simulink model "Telerobotic_System"  (R2020a)
settings: Solver=VariableStepAuto  StartTime=0.0  StopTime=10.0  RelTol=1e-3
values from neighbouring files (symbols this model uses):
  B = 1 / k_m    (= 0.0517063081696)    [Teleop_parameters.m]    (also in base.mat; base_no_attrito.mat = 0; ci_siamo.mat; force_control.mat)
  Be = 5    [Teleop_parameters.m]    (also in base.mat = 0.5; base_no_attrito.mat = 0.5; ci_siamo.mat; force_control.mat = 0.5)
  Bh = 0.02    [Teleop_parameters.m]    (also in base.mat; base_no_attrito.mat; ci_siamo.mat; force_control.mat)
  Fc_h = 5    [Teleop_parameters.m]    (also in base.mat; base_no_attrito.mat; ci_siamo.mat; force_control.mat)
  J = tau_m / k_m    (= 0.0629265770424)    [Teleop_parameters.m]    (also in base.mat; base_no_attrito.mat; ci_siamo.mat; force_control.mat)
  J_r = J + J * 0.5    (= 0.0943898655636)    [Teleop_parameters.m]    (also in base.mat; base_no_attrito.mat; ci_siamo.mat = 0.0629265770424; force_control.mat)
  Jh = 0.02    [Teleop_parameters.m]    (also in base.mat; base_no_attrito.mat; ci_siamo.mat; force_control.mat)
  k_m = 19.34    [Teleop_parameters.m]    (also in base.mat; base_no_attrito.mat; ci_siamo.mat; force_control.mat)
  k_s = 19.34    [Teleop_parameters.m]    (also in base.mat; base_no_attrito.mat; ci_siamo.mat; force_control.mat)
  Kc2v_m = 2    [Teleop_parameters.m]    (also in base.mat; base_no_attrito.mat; ci_siamo.mat; force_control.mat)
  Kc2v_s = 2    [Teleop_parameters.m]    (also in base.mat; base_no_attrito.mat; ci_siamo.mat; force_control.mat)
  Kd_h = 1    [Teleop_parameters.m]    (also in base.mat; base_no_attrito.mat; ci_siamo.mat = 10; force_control.mat)
  Kd_m = 1    [Teleop_parameters.m]    (also in base.mat; base_no_attrito.mat; ci_siamo.mat = 0.005; force_control.mat)
  Ke = 10    [Teleop_parameters.m]    (also in base.mat; base_no_attrito.mat; ci_siamo.mat; force_control.mat)
  Kp_h = 1.2    [Teleop_parameters.m]    (also in base.mat; base_no_attrito.mat; ci_siamo.mat = 10; force_control.mat)
  Kp_m = 1    [Teleop_parameters.m]    (also in base.mat; base_no_attrito.mat; ci_siamo.mat = 0.01; force_control.mat)
  Kt2c_m = 1.182    [Teleop_parameters.m]    (also in base.mat; base_no_attrito.mat; ci_siamo.mat; force_control.mat)
  Kt2c_s = 1.182    [Teleop_parameters.m]    (also in base.mat; base_no_attrito.mat; ci_siamo.mat; force_control.mat)
  Kv_fc = 30    [Teleop_parameters.m]    (also in base.mat = 0; base_no_attrito.mat = 0; ci_siamo.mat = 10; force_control.mat)
  lArm_m = 0.1    [Teleop_parameters.m]    (also in base.mat; base_no_attrito.mat; ci_siamo.mat; force_control.mat)
  lArm_s = 0.1    [Teleop_parameters.m]    (also in base.mat; base_no_attrito.mat; ci_siamo.mat; force_control.mat)
  maxCurrent_m = 4.5    [Teleop_parameters.m]    (also in base.mat; base_no_attrito.mat; ci_siamo.mat; force_control.mat)
  maxCurrent_s = 4.5    [Teleop_parameters.m]    (also in base.mat; base_no_attrito.mat; ci_siamo.mat; force_control.mat)
  qe = 5    [Teleop_parameters.m]    (also in base.mat; base_no_attrito.mat; ci_siamo.mat = 0.5; force_control.mat)
  tau_m = 1.217    [Teleop_parameters.m]    (also in base.mat; base_no_attrito.mat; ci_siamo.mat; force_control.mat)
  tau_s = 1.217    [Teleop_parameters.m]    (also in base.mat; base_no_attrito.mat; ci_siamo.mat; force_control.mat)
settings Model: Creator=gbagolin  LastModifiedBy=gbagolin

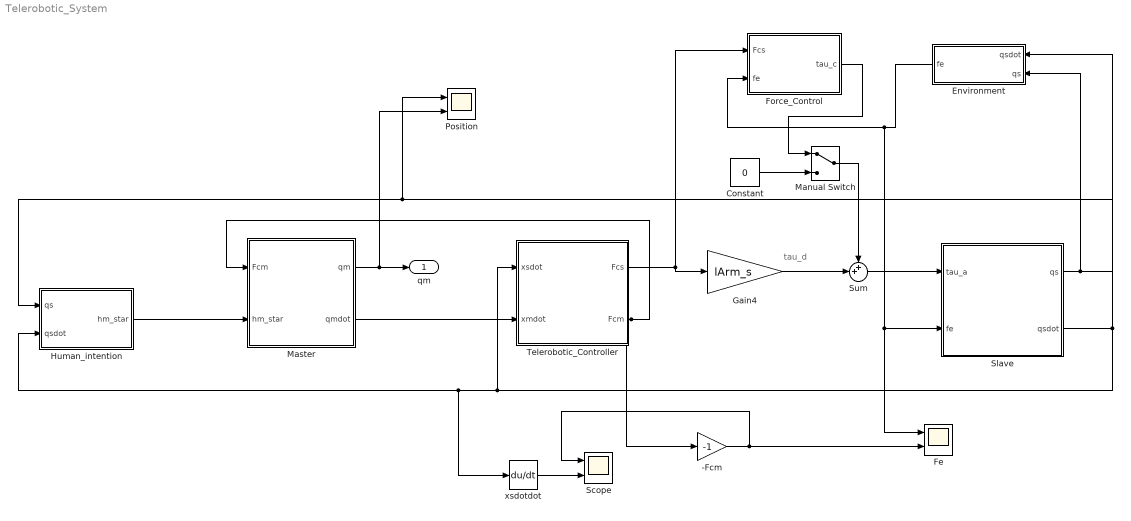
== system Telerobotic_System ==
  note: tau_d
  -Fcm : Gain  Gain=-1
  Constant : Constant  Value=0
  Environment : Subsystem
  Fe : Scope  NumInputPorts=2
  Force_Control : Subsystem
  Gain4 : Gain  Gain=lArm_s
  Human_intention : Subsystem
  Manual Switch : ManualSwitch
  Master : Subsystem
  Position : Scope  NumInputPorts=2
  Scope : Scope  NumInputPorts=2
  Slave : Subsystem
  Sum : Sum  Inputs=++|
  Telerobotic_Controller : Subsystem
  xsdotdot : Derivative  CoefficientInTFapproximation=0.001
  qm : Outport
  wires:
  Master/1(qm) -> Position/2, qm/1
  Master/2(qmdot) -> Telerobotic_Controller/2(xmdot)
  Telerobotic_Controller/2(Fcm) -> Master/1(Fcm), -Fcm/1
  Slave/1(qs) -> Environment/2(qs), Human_intention/1(qs), Position/1
  Human_intention/1(hm_star) -> Master/2(hm_star)
  Gain4/1 -> Sum/2
  Telerobotic_Controller/1(Fcs) -> Gain4/1, Force_Control/1(Fcs)
  Force_Control/1(tau_c) -> Manual Switch/1
  Sum/1 -> Slave/1(tau_a)
  Slave/2(qsdot) -> xsdotdot/1, Human_intention/2(qsdot), Telerobotic_Controller/1(xsdot), Environment/1(qsdot)
  Environment/1(fe) -> Fe/1, Slave/2(fe), Force_Control/2(fe)
  -Fcm/1 -> Scope/1, Fe/2
  Constant/1 -> Manual Switch/2
  Manual Switch/1 -> Sum/1
  xsdotdot/1 -> Scope/2

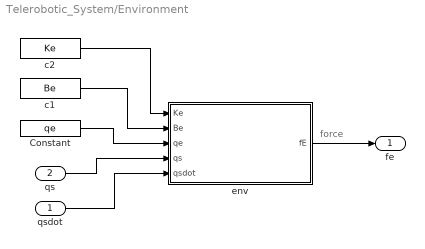
== system Telerobotic_System/Environment ==
  note: force
  qsdot : Inport
  qs : Inport  Port=2
  Constant : Constant  Value=qe  SampleTime=0
  c1 : Constant  Value=Be  SampleTime=0
  c2 : Constant  Value=Ke  SampleTime=0
  env : MATLAB Function  TreatAsAtomicUnit=on
  fe : Outport  VectorParamsAs1DForOutWhenUnconnected=off
  wires:
  Constant/1 -> env/3(qe)
  c1/1 -> env/2(Be)
  c2/1 -> env/1(Ke)
  qs/1 -> env/4(qs)
  qsdot/1 -> env/5(qsdot)
  env/1(fE) -> fe/1

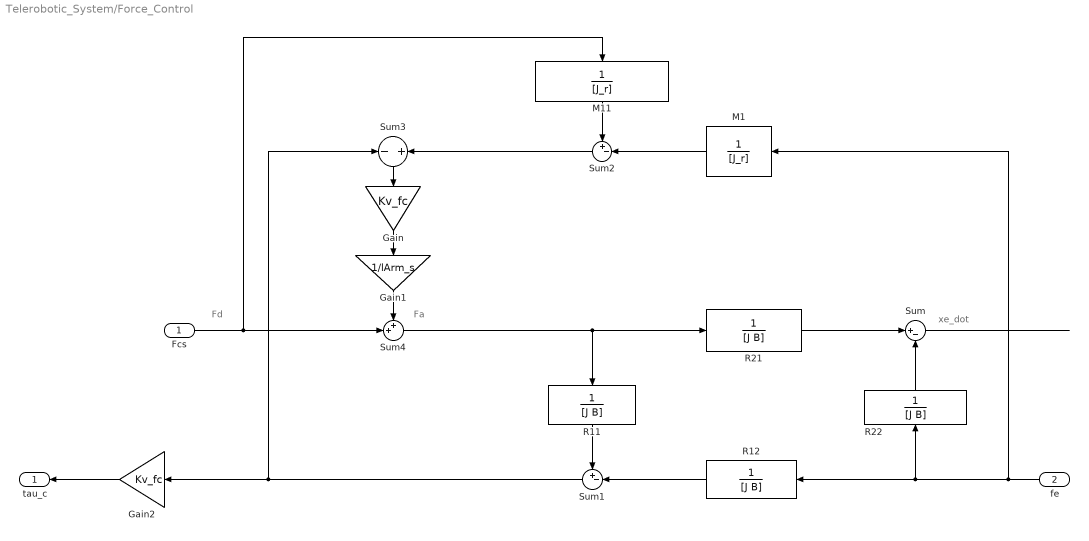
== system Telerobotic_System/Force_Control ==
  note: xe_dot
  note: Fa
  note: Fd
  Fcs : Inport
  fe : Inport  Port=2
  Gain : Gain  Gain=Kv_fc
  Gain1 : Gain  Gain=1/lArm_s
  Gain2 : Gain  Gain=Kv_fc
  M1 : TransferFcn  Denominator=[J_r]
  M11 : TransferFcn  Denominator=[J_r]
  R{11..12,21..22} (4 alike) : TransferFcn  Denominator=[J B]
  Sum : Sum  Inputs=|+-
  Sum1 : Sum  Inputs=+-|
  Sum2 : Sum  Inputs=+-|
  Sum3 : Sum  Inputs=-|+
  Sum4 : Sum  Inputs=++|
  tau_c : Outport
  wires:
  M1/1 -> Sum2/2
  M11/1 -> Sum2/1
  Gain/1 -> Gain1/1
  R21/1 -> Sum/1
  Sum4/1 -> R11/1, R21/1
  R11/1 -> Sum1/1
  Gain2/1 -> tau_c/1
  R12/1 -> Sum1/2
  Sum2/1 -> Sum3/2
  R22/1 -> Sum/2
  fe/1 -> R12/1, R22/1, M1/1
  Sum3/1 -> Gain/1
  Gain1/1 -> Sum4/1
  Fcs/1 -> M11/1, Sum4/2
  Sum1/1 -> Sum3/1, Gain2/1
  Sum/1 -> ?

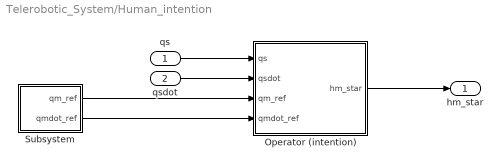
== system Telerobotic_System/Human_intention ==
  qs : Inport
  qsdot : Inport  Port=2
  Operator (intention) : Subsystem
  Subsystem : Subsystem
  hm_star : Outport
  wires:
  Subsystem/1(qm_ref) -> Operator (intention)/3(qm_ref)
  Subsystem/2(qmdot_ref) -> Operator (intention)/4(qmdot_ref)
  Operator (intention)/1(hm_star) -> hm_star/1
  qs/1 -> Operator (intention)/1(qs)
  qsdot/1 -> Operator (intention)/2(qsdot)

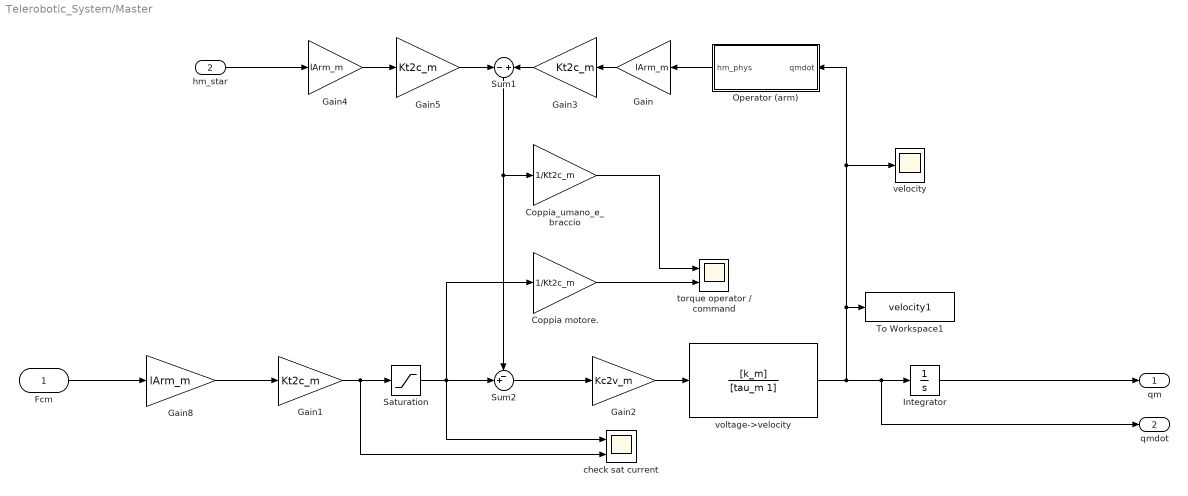
== system Telerobotic_System/Master ==
  Fcm : Inport
  hm_star : Inport  Port=2
  Coppia motore. : Gain  Gain=1/Kt2c_m
  Coppia_umano_e_braccio : Gain  Gain=1/Kt2c_m
  Gain : Gain  Gain=lArm_m
  Gain1 : Gain  Gain=Kt2c_m
  Gain2 : Gain  Gain=Kc2v_m
  Gain3 : Gain  Gain=Kt2c_m
  Gain4 : Gain  Gain=lArm_m
  Gain5 : Gain  Gain=Kt2c_m
  Gain8 : Gain  Gain=lArm_m
  Integrator : Integrator
  Operator (arm) : Subsystem
  Saturation : Saturate  UpperLimit=maxCurrent_m  LowerLimit=-maxCurrent_m
  Sum1 : Sum  Inputs=-+
  Sum2 : Sum  Inputs=-+|
  To Workspace1 : ToWorkspace  VariableName=velocity1  SaveFormat=Timeseries  SampleTime=-1
  check sat current : Scope  NumInputPorts=2
  torque operator / command : Scope  NumInputPorts=2
  velocity : Scope
  voltage->velocity : TransferFcn  Numerator=[k_m]  Denominator=[tau_m 1]
  qm : Outport
  qmdot : Outport  Port=2
  wires:
  Integrator/1 -> qm/1
  Sum2/1 -> Gain2/1
  Gain3/1 -> Sum1/2
  Gain2/1 -> voltage->velocity/1
  Gain1/1 -> check sat current/2, Saturation/1
  Coppia_umano_e_braccio/1 -> torque operator / command/1
  Coppia motore./1 -> torque operator / command/2
  voltage->velocity/1 -> velocity/1, Operator (arm)/1(qmdot), To Workspace1/1, qmdot/1, Integrator/1
  Gain8/1 -> Gain1/1
  Gain5/1 -> Sum1/1
  Operator (arm)/1(hm_phys) -> Gain/1
  Sum1/1 -> Sum2/1, Coppia_umano_e_braccio/1
  Saturation/1 -> Coppia motore./1, Sum2/2, check sat current/1
  Gain/1 -> Gain3/1
  Gain4/1 -> Gain5/1
  Fcm/1 -> Gain8/1
  hm_star/1 -> Gain4/1

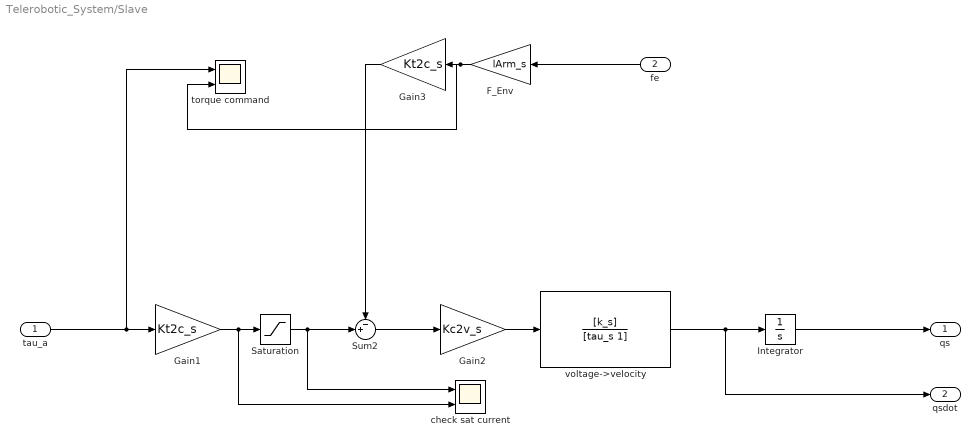
== system Telerobotic_System/Slave ==
  tau_a : Inport
  fe : Inport  Port=2
  F_Env : Gain  Gain=lArm_s
  Gain1 : Gain  Gain=Kt2c_s
  Gain2 : Gain  Gain=Kc2v_s
  Gain3 : Gain  Gain=Kt2c_s
  Integrator : Integrator
  Saturation : Saturate  UpperLimit=maxCurrent_s  LowerLimit=-maxCurrent_s
  Sum2 : Sum  Inputs=-+|
  check sat current : Scope  NumInputPorts=2
  torque command : Scope  NumInputPorts=2
  voltage->velocity : TransferFcn  Numerator=[k_s]  Denominator=[tau_s 1]
  qs : Outport
  qsdot : Outport  Port=2
  wires:
  fe/1 -> F_Env/1
  Integrator/1 -> qs/1
  Sum2/1 -> Gain2/1
  Saturation/1 -> Sum2/2, check sat current/1
  F_Env/1 -> torque command/2, Gain3/1
  Gain2/1 -> voltage->velocity/1
  voltage->velocity/1 -> qsdot/1, Integrator/1
  Gain1/1 -> check sat current/2, Saturation/1
  Gain3/1 -> Sum2/1
  tau_a/1 -> torque command/1, Gain1/1

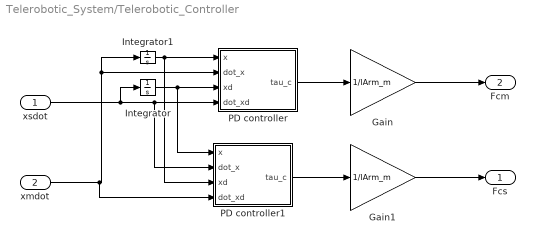
== system Telerobotic_System/Telerobotic_Controller ==
  xsdot : Inport
  xmdot : Inport  Port=2
  Gain : Gain  Gain=1/lArm_m
  Gain1 : Gain  Gain=1/lArm_m
  Integrator : Integrator
  Integrator1 : Integrator
  PD controller : Subsystem
  PD controller1 : Subsystem
  Fcs : Outport
  Fcm : Outport  Port=2
  wires:
  Integrator/1 -> PD controller1/1(x), PD controller/3(xd)
  Integrator1/1 -> PD controller1/3(xd), PD controller/1(x)
  PD controller1/1(tau_c) -> Gain1/1
  PD controller/1(tau_c) -> Gain/1
  xsdot/1 -> PD controller1/2(dot_x), PD controller/4(dot_xd), Integrator/1
  Gain1/1 -> Fcs/1
  Gain/1 -> Fcm/1
  xmdot/1 -> PD controller1/4(dot_xd), Integrator1/1, PD controller/2(dot_x)

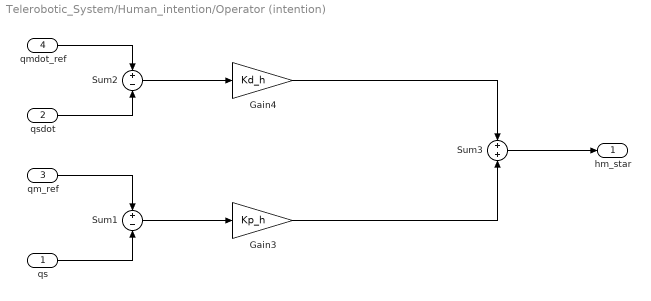
== system Telerobotic_System/Human_intention/Operator (intention) ==
  qs : Inport
  qsdot : Inport  Port=2
  qm_ref : Inport  Port=3
  qmdot_ref : Inport  Port=4
  Gain3 : Gain  Gain=Kp_h
  Gain4 : Gain  Gain=Kd_h
  Sum1 : Sum  Inputs=+|-
  Sum2 : Sum  Inputs=+|-
  Sum3 : Sum  Inputs=+|+
  hm_star : Outport  VectorParamsAs1DForOutWhenUnconnected=off
  wires:
  qs/1 -> Sum1/2
  qm_ref/1 -> Sum1/1
  qmdot_ref/1 -> Sum2/1
  Sum1/1 -> Gain3/1
  qsdot/1 -> Sum2/2
  Sum2/1 -> Gain4/1
  Gain4/1 -> Sum3/1
  Gain3/1 -> Sum3/2
  Sum3/1 -> hm_star/1

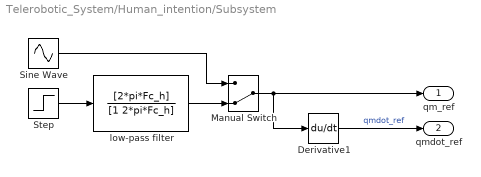
== system Telerobotic_System/Human_intention/Subsystem ==
  Derivative1 : Derivative  CoefficientInTFapproximation=0.001
  Manual Switch : ManualSwitch  CurrentSetting=0
  Sine Wave : Sin  SampleTime=0
  Step : Step  After=10  SampleTime=0
  low-pass filter : TransferFcn  Numerator=[2*pi*Fc_h]  Denominator=[1 2*pi*Fc_h]
  qm_ref : Outport
  qmdot_ref : Outport  Port=2
  wires:
  low-pass filter/1 -> Manual Switch/2
  Manual Switch/1 -> qm_ref/1, Derivative1/1
  Derivative1/1 -> qmdot_ref/1  "qmdot_ref"
  Step/1 -> low-pass filter/1
  Sine Wave/1 -> Manual Switch/1

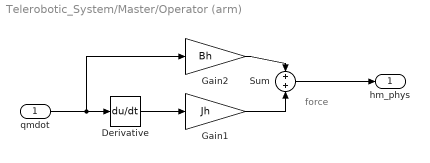
== system Telerobotic_System/Master/Operator (arm) ==
  note: force
  qmdot : Inport
  Derivative : Derivative  CoefficientInTFapproximation=0.001
  Gain1 : Gain  Gain=Jh
  Gain2 : Gain  Gain=Bh
  Sum : Sum  Inputs=+|+
  hm_phys : Outport  VectorParamsAs1DForOutWhenUnconnected=off
  wires:
  qmdot/1 -> Gain2/1, Derivative/1
  Sum/1 -> hm_phys/1
  Derivative/1 -> Gain1/1
  Gain2/1 -> Sum/1
  Gain1/1 -> Sum/2

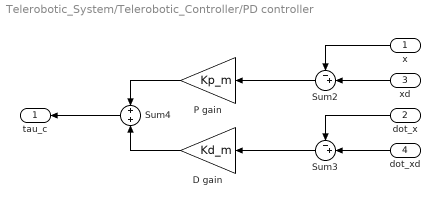
== system Telerobotic_System/Telerobotic_Controller/PD controller ==
  x : Inport
  dot_x : Inport  Port=2
  xd : Inport  Port=3
  dot_xd : Inport  Port=4
  D gain : Gain  Gain=Kd_m
  P gain : Gain  Gain=Kp_m
  Sum2 : Sum  Inputs=-+|
  Sum3 : Sum  Inputs=-+|
  Sum4 : Sum
  tau_c : Outport  VectorParamsAs1DForOutWhenUnconnected=off
  wires:
  D gain/1 -> Sum4/2
  dot_x/1 -> Sum3/1
  dot_xd/1 -> Sum3/2
  x/1 -> Sum2/1
  xd/1 -> Sum2/2
  Sum3/1 -> D gain/1
  P gain/1 -> Sum4/1
  Sum4/1 -> tau_c/1
  Sum2/1 -> P gain/1

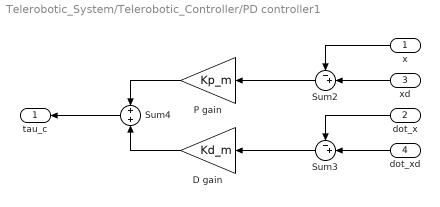
== system Telerobotic_System/Telerobotic_Controller/PD controller1 ==
  x : Inport
  dot_x : Inport  Port=2
  xd : Inport  Port=3
  dot_xd : Inport  Port=4
  D gain : Gain  Gain=Kd_m
  P gain : Gain  Gain=Kp_m
  Sum2 : Sum  Inputs=-+|
  Sum3 : Sum  Inputs=-+|
  Sum4 : Sum
  tau_c : Outport  VectorParamsAs1DForOutWhenUnconnected=off
  wires:
  D gain/1 -> Sum4/2
  dot_x/1 -> Sum3/1
  dot_xd/1 -> Sum3/2
  x/1 -> Sum2/1
  xd/1 -> Sum2/2
  Sum3/1 -> D gain/1
  P gain/1 -> Sum4/1
  Sum4/1 -> tau_c/1
  Sum2/1 -> P gain/1

== matlab function Telerobotic_System/Environment/env ==
  data: Ke input; Be input; qe input; qs input; fE output; qsdot input
function fE  = environment(Ke, Be, qe, qs, qsdot)
if qs > qe
   fE = Ke * (qs - qe) + Be * qsdot;
else
   fE = 0;
end
